simulink model "Practica6simulink"  (R2024a)
settings: Solver=VariableStepAuto  StartTime=0.0  StopTime=0.01  RelTol=1e-9
settings Model: Creator=52331  LastModifiedBy=52331

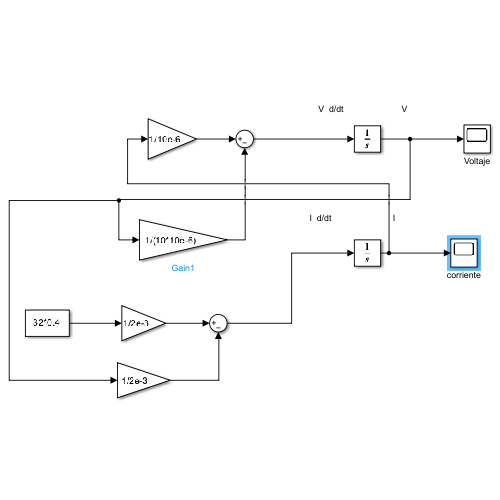
[thumbnail: Simulink's stored preview of the top-level diagram]
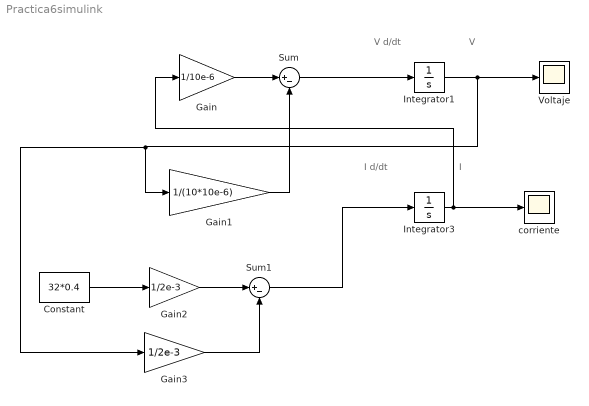
== system Practica6simulink ==
  note: V d/dt
  note: V
  note: I
  note: I d/dt
  Constant : Constant  Value=32*0.4
  Gain : Gain  Gain=1/10e-6
  Gain1 : Gain  Gain=1/(10*10e-6)
  Gain2 : Gain  Gain=1/2e-3
  Gain3 : Gain  Gain=1/2e-3
  Integrator1 : Integrator
  Integrator3 : Integrator
  Sum : Sum  Inputs=|+-
  Sum1 : Sum  Inputs=|+-
  Voltaje : Scope
  corriente : Scope
  wires:
  Integrator3/1 -> corriente/1, Gain/1
  Integrator1/1 -> Gain3/1, Gain1/1, Voltaje/1
  Gain1/1 -> Sum/2
  Gain/1 -> Sum/1
  Sum/1 -> Integrator1/1
  Constant/1 -> Gain2/1
  Gain2/1 -> Sum1/1
  Gain3/1 -> Sum1/2
  Sum1/1 -> Integrator3/1
